simulink model "lab6_OnlineClassifier"  (R2023a)
settings: Solver=FixedStepAuto  StartTime=0.0  StopTime=inf  FixedStep=1/30  RelTol=1e-3  EnableMultiTasking=on
values from neighbouring files (symbols this model uses):
  cc = zeros(NC,cd)    [lab6_HuMomentDescriptors.m]
  featuresRho = descripRho.Features    [lab5_buildDescriptors.m]
  featuresSqu = descripSqu.Features    [lab5_buildDescriptors.m]
  featuresTri = descripTri.Features    [lab5_buildDescriptors.m]
undefined symbols (not defined in the file or in its folder): coeff, none, videoinput
libraries: imaqlib x1, visionsources x1, visionsinks x1
settings Model: Creator=cardeira  LastModifiedBy=alexa
settings SolverCC: AlgebraicLoopSolver=TrustRegion
settings DataIOCC: LimitDataPoints=on  SaveFormat=Array  SignalLoggingSaveFormat=ModelDataLogs  ReturnWorkspaceOutputs=off
settings OptimizationCC: ExpressionDepthLimit=2147483647  LifeSpan=inf
settings DebuggingCC: UnderspecifiedInitializationDetection=Classic  MergeDetectMultiDrivingBlocksExec=none  SolverPrmCheckMsg=warning  FcnCallInpInsideContextMsg=warning  UnconnectedInputMsg=warning  UnconnectedOutputMsg=warning  UnconnectedLineMsg=warning  AllowSymbolicDim=off  StateNameClashWarn=warning  SFUnexpectedBacktrackingDiag=warning  SFNoUnconditionalDefaultTransitionDiag=warning  ArithmeticOperatorsInVariantConditions=warning
settings HardwareCC: ProdBitPerPointer=32  ProdBitPerSizeT=32  ProdBitPerPtrDiffT=32  ProdLargestAtomicFloat=None  ProdIntDivRoundTo=Undefined  ProdEndianess=Unspecified  ProdWordSize=32  ProdHWDeviceType=32-bit Generic
settings ModelReferenceCC: EnableRefExpFcnMdlSchedulingChecks=on  PropagateSignalLabelsOutOfModel=off
settings SFSimCC: SimUseLocalCustomCode=off  CustomCodeUndefinedFunction=UseInterfaceOnly
settings RTWCC: RTWUseLocalCustomCode=off  DLArmComputeVersion=19.05
settings CodeAppCC: StateflowObjectComments=on
settings GRTTargetCC: TargetLangStandard=C89/C90 (ANSI)  CombineOutputUpdateFcns=off  GRTInterface=on
settings ConfigComp: CovMetricSettings=dw  CovSaveCumulativeToWorkspaceVar=on  CovSaveSingleToWorkspaceVar=on  CovExternalEMLEnable=off  CovSFcnEnable=off

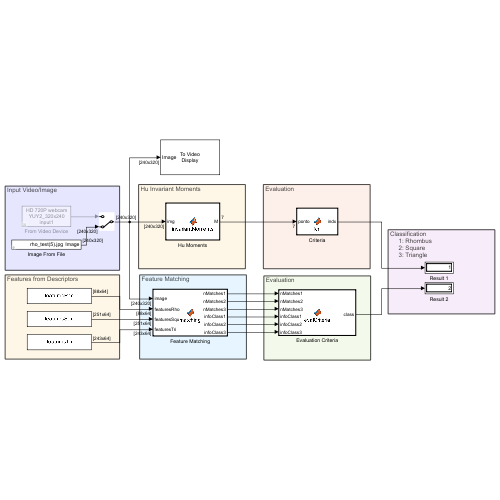
[thumbnail: Simulink's stored preview of the top-level diagram]
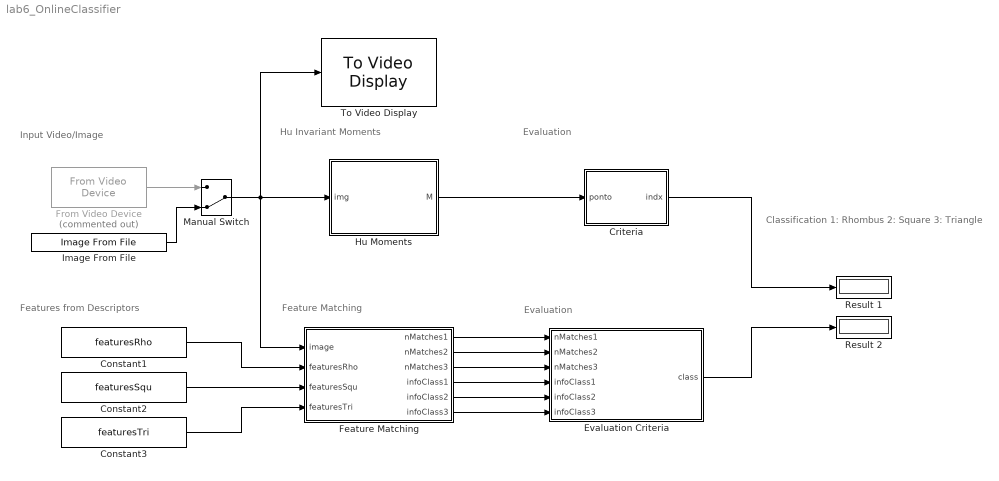
== system lab6_OnlineClassifier ==
  note: Input Video/Image
  note: Feature Matching
  note: Evaluation
  note: Features from Descriptors
  note: Hu Invariant Moments
  note: Classification
      |      1: Rhombus
      |      2: Square
      |      3: Triangle
  note: Evaluation
  " From Video Device " : imaqlib/From Video Device  Commented=on  DeviceMenu=(none)  Device=winvideo 1 (HD 720P webcam)  ObjConstructor=videoinput('winvideo', 1)  VideoFormatMenu=(none)  VideoFormat=YUY2_320x240  VideoSource=input1  ROIPosition=[0 0 240 320]  EnableHWTrigger=off  TriggerConfiguration=none/none  SampleTime=0.1  OutputPortsMode=One multidimensional signal  DataType=single  CanDoHWTrigger=no  ReturnedColorSpace=grayscale  BlockHandle=341.0026  ROIWidth=320  ROIHeight=240  ROIColumn=0  ROIRow=0  EngXMLPath=C:\Program Files\MATLAB\R2023a\toolbox\imaq\imaq\private  DevXMLPath=C:\ProgramData\MATLAB\SupportPackages\R2021a\toolbox\imaq\supportpackages\genericvideo\adaptor\win64  EngLibPath=C:\Program Files\MATLAB\R2023a\toolbox\imaq\imaqblks\imaqmex\win64  ColorSpace=grayscale  BayerSensorAlignment=grbg  ImaqMode=off
  " Image From File " : visionsources/Image From File  Tag=vipblks_nd  FileName=rho_test(5).jpg  Ts=0.1  imagePorts=One multidimensional signal  OutPortLabels=R|G|B  ImageDataType=single  sdImageDataType=uint(8)  Signed=on  WordLength=16  FractionLengthMode=User-defined  FractionLength=15
  Constant1 : Constant  Value=featuresRho  OutDataTypeStr=single
  Constant2 : Constant  Value=featuresSqu  OutDataTypeStr=single
  Constant3 : Constant  Value=featuresTri  OutDataTypeStr=single
  Criteria : MATLAB Function  TreatAsAtomicUnit=on
  Evaluation Criteria : MATLAB Function  TreatAsAtomicUnit=on
  Feature Matching : MATLAB Function  TreatAsAtomicUnit=on
  Hu Moments : MATLAB Function  InitFcn=load('HuMoments.mat')  TreatAsAtomicUnit=on
  Manual Switch : ManualSwitch  CurrentSetting=0
  Result 1 : Display
  Result 2 : Display
  To Video Display : visionsinks/To Video Display  windowSizeMode=Normal  openAtMdlStart=on  fullScreen=off  videoWindowX=1  videoWindowY=31  saveWindowSize=off  videoWindowWidth=958  videoWindowHeight=1008  inputColorFormat=RGB  inputType=Obsolete  imagePorts=One multidimensional signal  OutputDevice=On-screen video monitor  dataOrg=Column-major  isWindowOpen=off
  wires:
  Manual Switch/1 -> Hu Moments/1(img), To Video Display/1, Feature Matching/1(image)
  " From Video Device "/1 -> Manual Switch/1
  " Image From File "/1 -> Manual Switch/2
  Constant1/1 -> Feature Matching/2(featuresRho)
  Feature Matching/3(nMatches3) -> Evaluation Criteria/3(nMatches3)
  Feature Matching/2(nMatches2) -> Evaluation Criteria/2(nMatches2)
  Feature Matching/1(nMatches1) -> Evaluation Criteria/1(nMatches1)
  Feature Matching/4(infoClass1) -> Evaluation Criteria/4(infoClass1)
  Feature Matching/5(infoClass2) -> Evaluation Criteria/5(infoClass2)
  Feature Matching/6(infoClass3) -> Evaluation Criteria/6(infoClass3)
  Constant2/1 -> Feature Matching/3(featuresSqu)
  Constant3/1 -> Feature Matching/4(featuresTri)
  Hu Moments/1(M) -> Criteria/1(ponto)
  Criteria/1(indx) -> Result 1/1
  Evaluation Criteria/1(class) -> Result 2/1

== matlab function lab6_OnlineClassifier/Feature Matching ==
  data: image input; nMatches1 output; featuresRho input; featuresSqu input; featuresTri input; nMatches2 output; nMatches3 output; infoClass1 output; infoClass2 output; infoClass3 output
function [nMatches1, nMatches2, nMatches3, infoClass1, infoClass2, infoClass3] = matching(image, featuresRho, featuresSqu, featuresTri)
% Include additional functions
coder.extrinsic('detectSURFFeatures');
coder.extrinsic('detectHarrisFeatures');
coder.extrinsic('detectBRISKFeatures');
coder.extrinsic('detectFASTFeatures');
coder.extrinsic('detectORBFeatures');
coder.extrinsic('extractFeatures');
coder.extrinsic('matchFeatures');

% Initialize output variables as double
nMatches1 = double(0);
nMatches2 = double(0);
nMatches3 = double(0);
infoClass1 = double(0);
infoClass2 = double(0);
infoClass3 = double(0);

% ---------------- EDIT THE CODE HERE ---------------- %

ptsClassify = detectSURFFeatures(image);
[featClassify, ~] = extractFeatures(image, ptsClassify);

% Feature matching
matchedPairs1 = matchFeatures((featuresRho), featClassify);
matchedPairs2 = matchFeatures((featuresSqu), featClassify);
matchedPairs3 = matchFeatures((featuresTri), featClassify);

% ---------------- CHOOSE THE OUTPUT ---------------- %
nMatches1 = length(matchedPairs1);
nMatches2 = length(matchedPairs2);
nMatches3 = length(matchedPairs3);
infoClass1 = 0;
infoClass2 = 0;
infoClass3 = 0;
end

== matlab function lab6_OnlineClassifier/Criteria ==
  data: ponto input double; indx output; coeff parameter double; cc parameter double
function indx = fcn(ponto,coeff,cc)
%#codegen

coder.extrinsic('pdist2');

protate=round(ponto'*coeff*10000)/10000;
protate2d=protate(1,1:size(cc,2));   % redução da dimensão

distancias=zeros(length(cc),1);
for i=1:length(cc)
    dist=pdist2(cc(i,:),protate2d);
    distancias(i)=dist;
end
[~,indx]=min(distancias);

% try a minimum acceptable distance in order to reject other pieces not
% belonging to the expected classes. (these pieces should be classified as
% 0)

== matlab function lab6_OnlineClassifier/Evaluation Criteria ==
  data: nMatches1 input; class output; nMatches2 input; nMatches3 input; infoClass1 input; infoClass2 input; infoClass3 input
function class = evalCriteria(nMatches1, nMatches2, nMatches3, infoClass1, infoClass2, infoClass3)
% ---------------- EDIT THE CODE HERE ---------------- %
result1 = nMatches1;
result2 = nMatches2;
result3 = nMatches3;

% ---------------- CHOOSE THE OUTPUT ---------------- %
maxResult = max([result1, result2, result3]);
if maxResult == result1
    class = 1;
elseif maxResult == result2
    class = 2;
elseif maxResult == result3
    class = 3;
else
    class = 0;
end

end

== matlab function lab6_OnlineClassifier/Hu Moments ==
  data: img input; M output double
function M  = invariantMoments(img)

% Automatic binarization
A=imbinarize(img);
A=imcomplement(A);
coder.extrinsic('HuInvariantMoments');
outvar=HuInvariantMoments(A);

y1=coder.nullcopy(zeros(7,1)); % ver nota 
M=double(y1);
M=outvar;
